simulink model "controlador_chr_simulink"  (R2022b)
settings: Solver=VariableStepAuto  StartTime=0.0  StopTime=250  RelTol=1e-3
settings Model: Creator=fabio  LastModifiedBy=fabio

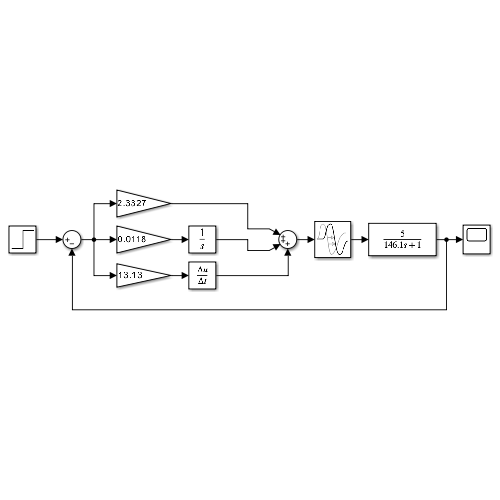
[thumbnail: Simulink's stored preview of the top-level diagram]
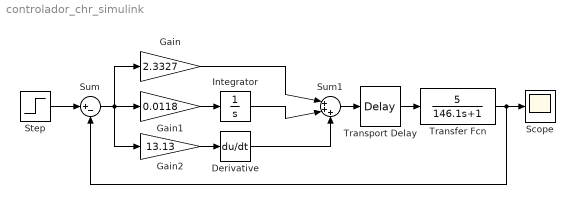
== system controlador_chr_simulink ==
  Derivative : Derivative
  Gain : Gain  Gain=2.3327
  Gain1 : Gain  Gain=0.0118
  Gain2 : Gain  Gain=13.13
  Integrator : Integrator
  Scope : Scope
  Step : Step  Time=0  After=4  SampleTime=0
  Sum : Sum  Inputs=|+-
  Sum1 : Sum  Inputs=|+++
  Transfer Fcn : TransferFcn  Numerator=[5]  Denominator=[146.1 1]
  Transport Delay : TransportDelay  DelayTime=11.9
  wires:
  Transport Delay/1 -> Transfer Fcn/1
  Transfer Fcn/1 -> Scope/1, Sum/2
  Step/1 -> Sum/1
  Sum1/1 -> Transport Delay/1
  Gain/1 -> Sum1/1
  Integrator/1 -> Sum1/2
  Derivative/1 -> Sum1/3
  Gain1/1 -> Integrator/1
  Gain2/1 -> Derivative/1
  Sum/1 -> Gain2/1, Gain/1, Gain1/1
